simulink model "MODEL_NA_SILNIK_PID"  (R2019b)
settings: Solver=FixedStepAuto  StartTime=0.0  StopTime=inf  RelTol=1e-3  EnableMultiTasking=on
undefined symbols (not defined in the file or in its folder): DiscIntNeverNeededParam, magnitude
libraries: simulink x3, embdlinuxlib x2, dspswit3 x2, raspberrypilib x1
settings Model: SILPILModeSetting=veronly  ExtModeTrigDuration=2  Creator=damia  LastModifiedBy=damia
settings SolverCC: PositivePriorityOrder=on
settings OptimizationCC: EnhancedBackFolding=on  PassReuseOutputArgsAs=Individual arguments  ZeroExternalMemoryAtStartup=off  ZeroInternalMemoryAtStartup=off  MaxStackSize=64  OptimizeBlockOrder=speed  DifferentSizesBufferReuse=on  OptimizationCustomize=off  EfficientTunableParamExpr=on
settings DebuggingCC: ParameterTunabilityLossMsg=error
settings HardwareCC: ProdBitPerPointer=32  ProdBitPerSizeT=32  ProdBitPerPtrDiffT=32  ProdLargestAtomicInteger=Long  ProdLargestAtomicFloat=Double  ProdWordSize=32  ProdLongLongMode=on  ProdHWDeviceType=ARM Compatible->ARM Cortex  UseEmbeddedCoderFeatures=off  UseSimulinkCoderFeatures=off
settings RTWCC: SystemTargetFile=ert.tlc  HardwareBoard=Raspberry Pi  TLCOptions="-aInlineSetEventsForThisBaseRateFcn=TLC_FALSE -aSuppressMultiTaskScheduler=TLC_FALSE  -aRateBasedStepFcn=0"  TemplateMakefile=ert_default_tmf  RTWVerbose=off  Toolchain=GNU GCC Raspberry Pi  BuildConfiguration=Faster Runs  IncludeHyperlinkInReport=on
settings CodeAppCC: ForceParamTrailComments=on  OperatorAnnotations=on  SimulinkDataObjDesc=on  SFDataObjDesc=on  InsertBlockDesc=on
settings ERTTargetCC: SupportContinuousTime=on  SupportNonInlinedSFcns=on  SupportVariableSizeSignals=on  ERTSrcFileBannerTemplate=codertarget_code_template.cgt  ERTHdrFileBannerTemplate=codertarget_code_template.cgt  ERTDataSrcFileTemplate=codertarget_code_template.cgt  ERTDataHdrFileTemplate=codertarget_code_template.cgt

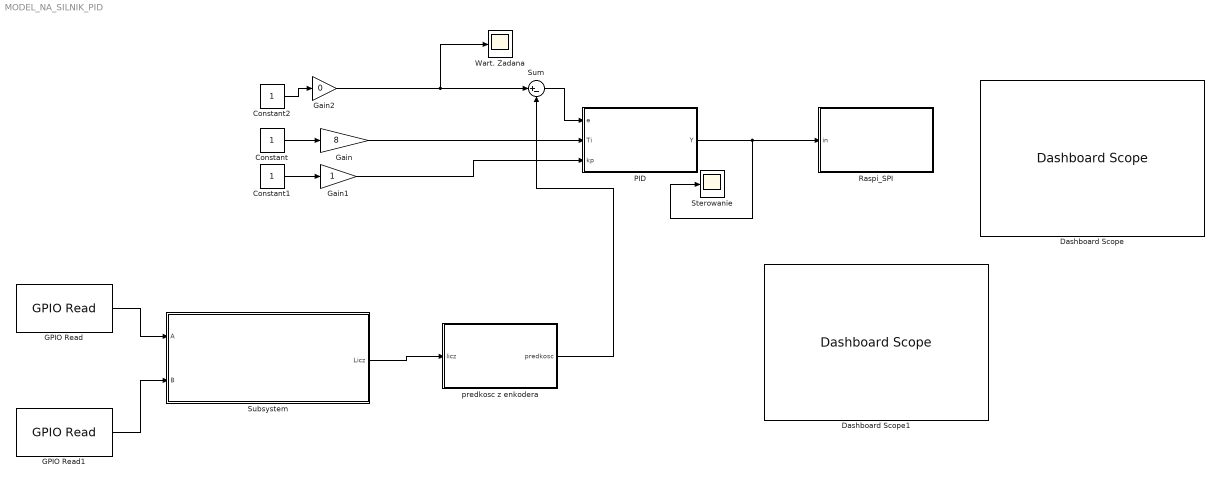
== system MODEL_NA_SILNIK_PID ==
  Constant : Constant
  Constant1 : Constant
  Constant2 : Constant
  Dashboard Scope : DashboardScope
  Dashboard Scope1 : DashboardScope
  GPIO Read : embdlinuxlib/GPIO Read  board=Pi 3 Model B  gpio=14  internalResistor=Off  sampleTime=.01  direction=Input  blockPlatform=Raspberry Pi
      settings: SourceProductName=Simulink Support Package for Raspberry Pi Hardware  SourceProductBaseCode=RASPPI
  GPIO Read1 : embdlinuxlib/GPIO Read  board=Pi 3 Model B  gpio=18  internalResistor=Off  sampleTime=.01  direction=Input  blockPlatform=Raspberry Pi
      settings: SourceProductName=Simulink Support Package for Raspberry Pi Hardware  SourceProductBaseCode=RASPPI
  Gain : Gain  Gain=8
  Gain1 : Gain
  Gain2 : Gain  Gain=0
  PID : Subsystem
  Raspi_SPI : Subsystem
  Sterowanie : Scope
  Subsystem : Subsystem
  Sum : Sum  Inputs=|+-
  Wart. Zadana : Scope
  predkosc z enkodera : Subsystem
  wires:
  Gain1/1 -> PID/3(kp)
  Sum/1 -> PID/1("e ")
  Subsystem/1(Licz) -> predkosc z enkodera/1("licz ")
  GPIO Read1/1 -> Subsystem/2(B)
  GPIO Read/1 -> Subsystem/1(A)
  predkosc z enkodera/1("predkosc ") -> Sum/2
  Constant/1 -> Gain/1
  Constant2/1 -> Gain2/1
  Gain2/1 -> Wart. Zadana/1, Sum/1
  Gain/1 -> PID/2(Ti)
  Constant1/1 -> Gain1/1
  PID/1(Y) -> Raspi_SPI/1("in "), Sterowanie/1

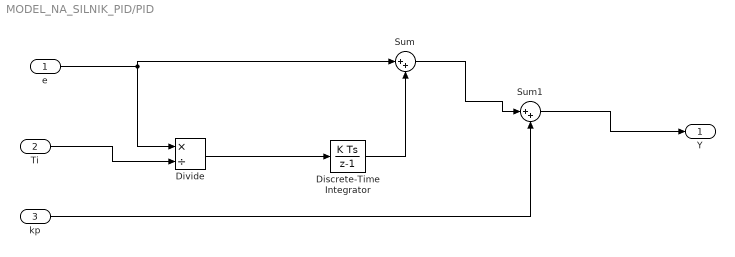
== system MODEL_NA_SILNIK_PID/PID ==
  "e " : Inport
  Ti : Inport  Port=2
  kp : Inport  Port=3
  Discrete-Time Integrator : DiscreteIntegrator  SampleTime=0.01  ICPrevOutput=DiscIntNeverNeededParam  ICPrevScaledInput=DiscIntNeverNeededParam
  Divide : Product  Inputs=*/
  Sum : Sum  Inputs=|++
  Sum1 : Sum  Inputs=|++
  Y : Outport
  wires:
  "e "/1 -> Sum/1, Divide/1
  Ti/1 -> Divide/2
  Divide/1 -> Discrete-Time Integrator/1
  Discrete-Time Integrator/1 -> Sum/2
  Sum/1 -> Sum1/1
  Sum1/1 -> Y/1
  kp/1 -> Sum1/2

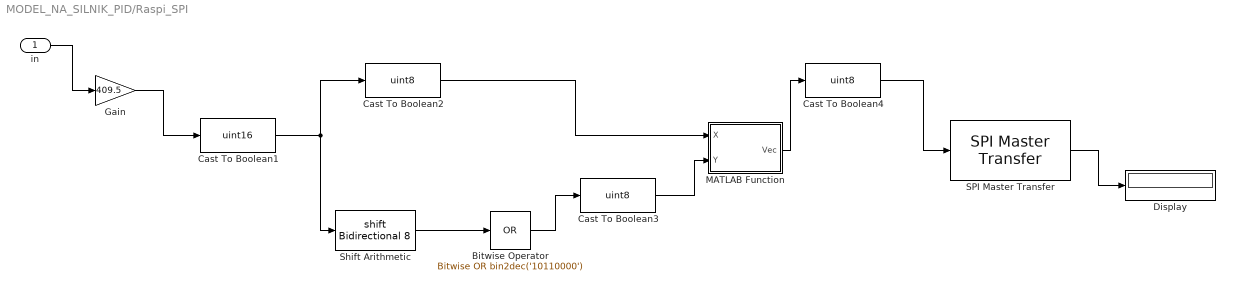
== system MODEL_NA_SILNIK_PID/Raspi_SPI ==
  "in " : Inport
  Bitwise Operator : simulink/Logic and Bit Operations/Bitwise Operator  logicop=OR  UseBitMask=on  BitMask=bin2dec('10110000')  BitMaskRealWorld=Real World Value
  Cast To Boolean1 : DataTypeConversion  OutDataTypeStr=uint16
  Cast To Boolean2 : DataTypeConversion  OutDataTypeStr=uint8
  Cast To Boolean3 : DataTypeConversion  OutDataTypeStr=uint8
  Cast To Boolean4 : DataTypeConversion  OutDataTypeStr=uint8
  Display : Display
  Gain : Gain  Gain=409.5
  MATLAB Function : MATLAB Function  TreatAsAtomicUnit=on
  SPI Master Transfer : raspberrypilib/SPI Master Transfer  Priority=1  BoardProperty=Pi 3 Model B  SPIModule=uint32(0)  Mode=Master  BusSpeed=1000000  Pin=SPI0_CE0  FirstBitToTransfer=Most significant bit (MSB)  ClockMode=0  BlockFunction=Transfer  RegisterAddress=0  OutputDataType=int8  OutputDataLength=1
      settings: SourceProductName=Simulink Support Package for Raspberry Pi Hardware  SourceProductBaseCode=RASPPI
  Shift Arithmetic : ArithShift  BitShiftNumber=8
  wires:
  SPI Master Transfer/1 -> Display/1
  MATLAB Function/1(Vec) -> Cast To Boolean4/1
  Cast To Boolean2/1 -> MATLAB Function/1(X)
  Shift Arithmetic/1 -> Bitwise Operator/1
  Bitwise Operator/1 -> Cast To Boolean3/1
  Cast To Boolean4/1 -> SPI Master Transfer/1
  Cast To Boolean3/1 -> MATLAB Function/2(Y)
  Cast To Boolean1/1 -> Cast To Boolean2/1, Shift Arithmetic/1
  Gain/1 -> Cast To Boolean1/1
  "in "/1 -> Gain/1

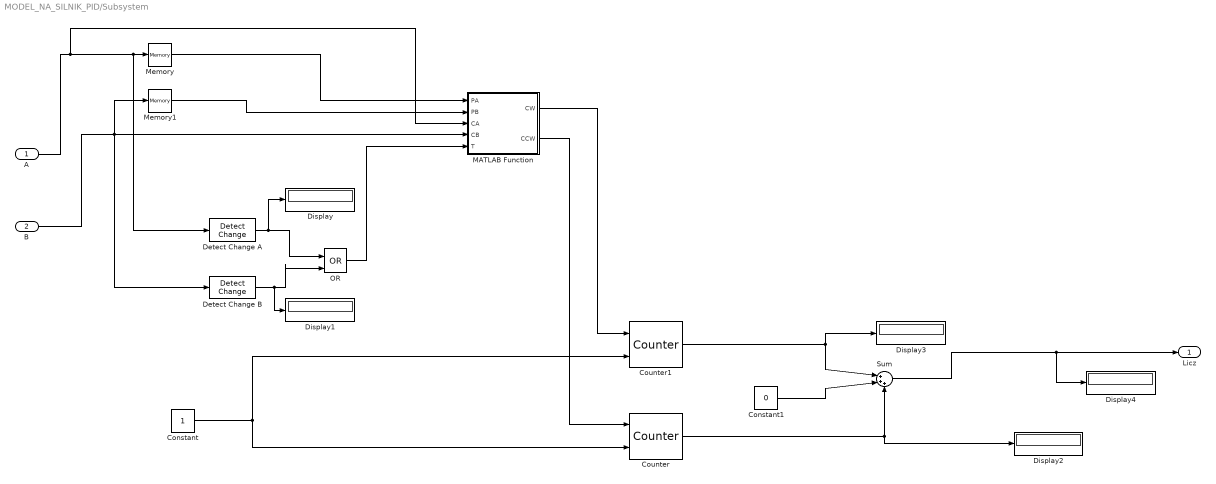
== system MODEL_NA_SILNIK_PID/Subsystem ==
  A : Inport
  B : Inport  Port=2
  Constant : Constant
  Constant1 : Constant  Value=0
  Counter : dspswit3/Counter  Direction=Up  CountEvent=Rising edge  CounterSize=User defined  MaxCount=1024  InitialCount=0  Output=Count  HitValue=0  ResetInput=on  SamplesPerFrame=1  Ts=1  CntDtype=double  HitDtype=Logical
  Counter1 : dspswit3/Counter  Direction=Up  CountEvent=Rising edge  CounterSize=User defined  MaxCount=1024  InitialCount=0  Output=Count  HitValue=0  ResetInput=on  SamplesPerFrame=1  Ts=1  CntDtype=double  HitDtype=Logical
  Detect Change A : simulink/Logic and Bit Operations/Detect Change  vinit=0  OutDataTypeStr=boolean
  Detect Change B : simulink/Logic and Bit Operations/Detect Change  vinit=0  OutDataTypeStr=boolean
  Display{,1..4} (5 alike) : Display
  MATLAB Function : MATLAB Function  TreatAsAtomicUnit=on
  Memory : Memory
  Memory1 : Memory
  OR : Logic  Operator=OR  IconShape=distinctive  AllPortsSameDT=off  OutDataTypeStr=boolean
  Sum : Sum  Inputs=|+++
  Licz : Outport
  wires:
  A/1 -> MATLAB Function/3(CA), Detect Change A/1, Memory/1
  B/1 -> MATLAB Function/4(CB), Detect Change B/1, Memory1/1
  Detect Change A/1 -> Display/1, OR/1
  Detect Change B/1 -> Display1/1, OR/2
  OR/1 -> MATLAB Function/5(T)
  Memory/1 -> MATLAB Function/1(PA)
  Memory1/1 -> MATLAB Function/2(PB)
  MATLAB Function/2(CCW) -> Counter/1
  MATLAB Function/1(CW) -> Counter1/1
  Constant/1 -> Counter1/2, Counter/2
  Constant1/1 -> Sum/2
  Counter/1 -> Display2/1, Sum/3
  Counter1/1 -> Sum/1, Display3/1
  Sum/1 -> Display4/1, Licz/1

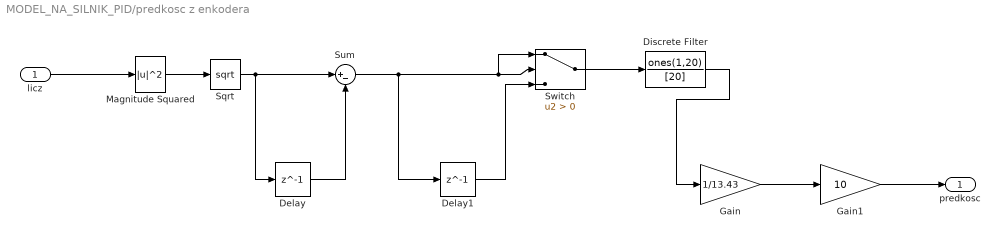
== system MODEL_NA_SILNIK_PID/predkosc z enkodera ==
  "licz " : Inport
  Delay : Delay  DelayLength=1  InitialCondition=0
  Delay1 : Delay  DelayLength=1  InitialCondition=0
  Discrete Filter : DiscreteFilter  Numerator=ones(1,20)  Denominator=[20]
  Gain : Gain  Gain=1/13.43
  Gain1 : Gain  Gain=10
  Magnitude Squared : Math  Operator=magnitude^2  SignedPower=off  SaturateOnIntegerOverflow=on
  Sqrt : Sqrt  IntermediateResultsDataTypeStr=double  SaturateOnIntegerOverflow=on
  Sum : Sum  Inputs=|+-
  Switch : Switch  Criteria=u2 > Threshold
  "predkosc " : Outport
  wires:
  "licz "/1 -> Magnitude Squared/1
  Magnitude Squared/1 -> Sqrt/1
  Sqrt/1 -> Delay/1, Sum/1
  Delay/1 -> Sum/2
  Sum/1 -> Switch/1, Switch/2, Delay1/1
  Delay1/1 -> Switch/3
  Switch/1 -> Discrete Filter/1
  Discrete Filter/1 -> Gain/1
  Gain/1 -> Gain1/1
  Gain1/1 -> "predkosc "/1

== matlab function MODEL_NA_SILNIK_PID/Subsystem/MATLAB Function ==
  data: PA input; CW output; PB input; CCW output; CA input; CB input; T input
function [CW,CCW] = encoder(PA,PB,CA,CB,T)

% persistent counter;
% if isempty(counter)
% counter = 0;
% end
% persistent aLastState;
% if isempty(aLastState)
% aLastState = a;
% end
% % 
% % out = aLastState
% % while(1)
%     aState = a;
%     bState = b;
%     if(aState ~= aLastState)
%         bstate = b;
%     end
%     if(bState ~=aState)
%         counter = counter+1;
%     else
%         counter = counter - 1;
%     end
%      out = counter;
%     aLastState = aState;
% end

CW = NaN; CCW = NaN;
if(T==1)
    if PA == 0
        if PB == 0
        if CA == 0 && CB == 1  %0001
            CW = 1;
            CCW = 0;
        elseif CA == 1 && CB == 0 %0010
            CW = 0;
            CCW = 1;
        end
    elseif PB == 1
        if CA == 1 && CB == 1 %0111
            CW=1;
            CCW=0;
        elseif CA == 0 && CB == 0 %0100
            CW = 0;
            CCW = 1;
        end
    end
elseif PA == 1
    if PB == 1
        if CA == 1 && CB == 0  % 1110
            CW = 1;
            CCW = 0;
        elseif CA == 0 && CB == 1  %1101
            CW = 0;
            CCW = 1;
        end
        
    elseif PB == 0 
        if CA == 0 && CB == 0  % 1000
            CW = 1; 
            CCW = 0;
        elseif CA == 1 && CB == 1 %1011
            CW = 0; 
            CCW = 1;
        end
    end
end
end
end

== matlab function MODEL_NA_SILNIK_PID/Raspi_SPI/MATLAB Function ==
  data: X input; Vec output; Y input
function Vec = Vector(X, Y)

% myPI = raspi();
Vec = [Y X];
% mySPI = spidev(myPI,'CE0');
% out = writeRead(mySPI,[Vec]);
